simulink model "State_Feedback_PIL_Simulation"  (R2021b)
settings: Solver=FixedStepAuto  StartTime=0.0  StopTime=10.0  RelTol=1e-3  EnableMultiTasking=on
undefined symbols (not defined in the file): den_d, num_d, Ts
settings Model: SILPILSystemUnderTest=refmodels  ExtModeTrigDuration=10  Creator=UTENTE  LastModifiedBy=UTENTE
settings OptimizationCC: EnhancedBackFolding=on  PassReuseOutputArgsAs=Individual arguments  ZeroExternalMemoryAtStartup=off  ZeroInternalMemoryAtStartup=off  MaxStackSize=64  OptimizeBlockOrder=speed  DifferentSizesBufferReuse=on  OptimizationCustomize=off  EfficientTunableParamExpr=on
settings DebuggingCC: ParameterTunabilityLossMsg=error
settings HardwareCC: ProdBitPerPointer=32  ProdBitPerSizeT=32  ProdBitPerPtrDiffT=32  ProdLargestAtomicInteger=Long  ProdLargestAtomicFloat=Double  ProdWordSize=32  ProdLongLongMode=on  ProdHWDeviceType=ARM Compatible->ARM Cortex
settings SFSimCC: MATLABDynamicMemAlloc=off
settings RTWCC: Description=Embedded Coder  SystemTargetFile=ert.tlc  HardwareBoard=STM32 Nucleo F401RE  TemplateMakefile=ert_default_tmf  Toolchain=GNU Tools for ARM Embedded Processors  CodeExecutionProfiling=on
settings CodeAppCC: ForceParamTrailComments=on  IgnoreCustomStorageClasses=off  OperatorAnnotations=on  SimulinkDataObjDesc=on  SFDataObjDesc=on  InsertBlockDesc=on
settings ERTTargetCC: ExtModeTransport=3  ExtModeStaticAlloc=on  ExtModeStaticAllocSize=2000  ExtModeMexFile=ext_xcp  ExtModeIntrfLevel=Level2 - Open

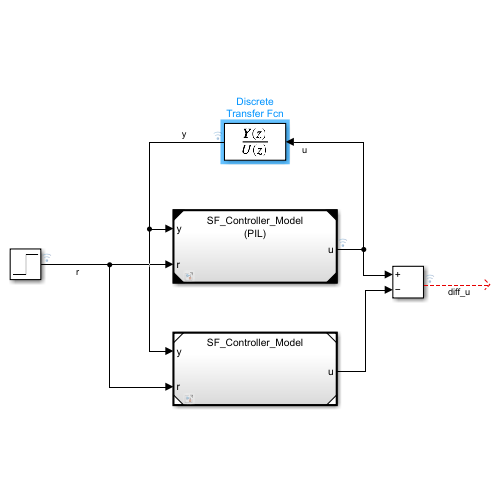
[thumbnail: Simulink's stored preview of the top-level diagram]
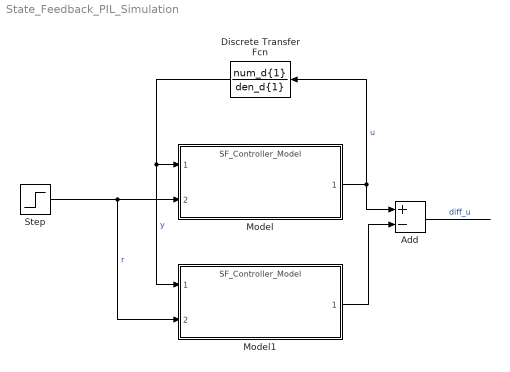
== system State_Feedback_PIL_Simulation ==
  Add : Sum  Inputs=+-
  Discrete Transfer Fcn : DiscreteTransferFcn  Numerator=num_d{1}  Denominator=den_d{1}  SampleTime=Ts
  Model : ModelReference  ModelNameDialog=SF_Controller_Model.slx  SimulationMode=Processor-in-the-loop (PIL)  ModelReferenceVersion=1.6
  Model1 : ModelReference  ModelNameDialog=SF_Controller_Model.slx  SimulationMode=Normal  ModelReferenceVersion=1.6
  Step : Step  After=125  SampleTime=Ts
  wires:
  Step/1 -> Model1/2, Model/2  "r"
  Discrete Transfer Fcn/1 -> Model1/1, Model/1  "y"
  Model1/1 -> Add/2
  Model/1 -> Discrete Transfer Fcn/1, Add/1  "u"
  Add/1 -> ?  "diff_u"
